simulink model "acc_with_sensor"  (R2021b)
settings: Solver=FixedStepAuto  StartTime=0.0  StopTime=206  FixedStep=0.0005  RelTol=1e-3
InitFcn:
  | G=9.81;
  | m=1660;
  | rw=0.325;
  | Caf=74070;
  | Car=58525;
  | Iz=2778.5;
  | d = 1.502;
  | lf =1.1135;
  | lr =1.5065;
  | L = 2.62;
  | kph2mps=1/3.6;
values from neighbouring files (symbols this model uses):
  Leftdis_PV_switch = 2    [acc_plot_backup.m]
  s_path = [0 1.10508939428 2.2141958029 3.32141571172 4.42705301151 5.53154548532 6.63517443471 7.73808041313 8.84055018688 9.94289959674 11.0453539299 12.1480581097 ... (1001 elements, 1001x1)]    [200_100radius.mat]    (also in LV_Clothoid_S_Turn_path.mat = [0 0.966832089581 1.93621320584 2.90214024471 3.86476766313 ; NEDC_path.mat = [0 0.414605943146 0.832514087334 1.25401518562 1.68216660344; Straight_East_into_curve.mat = [0 1.65770560069 3.32192925577 4.98420060507 6.64484613518 8; acc_plot_backup.m = Station_HV_m)
  X_path = [0 1.10508939428 2.2141958029 3.32141571172 4.42705301151 5.53154548532 6.63517443471 7.73808041313 8.84055018688 9.94289959674 11.0453539299 12.1480581097 ... (1001 elements, 1001x1)]    [200_100radius.mat]    (also in LV_Clothoid_S_Turn_path.mat = [-10 -9.03316791042 -8.06378679416 -7.09785975529 -6.1352323; NEDC_path.mat = [0 0.414605943146 0.832514087334 1.25401518562 1.68216660344; Straight_East_into_curve.mat = [0 1.65770560069 3.32192925577 4.98420060507 6.64484613518 8; acc_plot_backup.m = X_HV_m)
  Y_path = [0 -1.70364610795e-18 -7.41532896709e-18 1.46822109542e-17 4.74557362791e-17 6.12980216762e-17 9.25043977736e-17 1.24088240159e-16 1.5099156923e-16 1.7058517853e-16 1.90629227614e-16 2.09673434424e-16 ... (1001 elements, 1001x1)]    [200_100radius.mat]    (also in LV_Clothoid_S_Turn_path.mat = [0 -8.46153035536e-19 5.07382551045e-18 2.07356032218e-17 3.; NEDC_path.mat = [0 -3.50680326162e-18 -2.14111304971e-18 3.38197671014e-18 3; Straight_East_into_curve.mat = [0 1.29197709199e-18 2.81882429322e-18 3.49020462564e-17 6.7; acc_plot_backup.m = Y_HV_m)
undefined symbols (not defined in the file or in its folder): C_TICK_TIME_S, Cut_in_Secenary_flg, ENUM_ACCSTATE_DISABLED, ENUM_ACCSTATE_OFF, ENUM_ACCSTATE_STANDBY, FALSE, KVDI_ACCLongPressTime_ms, KVDI_ACCMaxActSpeed_kph, KVDI_ACCSetSpdIntial_kph, KVDI_ACCSpdLargeChange_kph, KVDI_LongPressConTime_ms, ONE_FLOAT, ONE_INT, raptor_xcp_function, T, TRUE, UseTTC_switch, ZERO_FLOAT, ZERO_INT
libraries: ADASLibrary x29, simulink x22, Raptor_lib x11, dspstat3 x6, simulink_extras x6, Solver_SF x1, mpclib x1
(part 8 of 9)

== system acc_with_sensor/Relative_Dynamic/Subsystem2/Subsystem ==
  In1 : Inport
  Abs : Abs
  Constant : Constant  Value=0.1
  Switch : Switch  Criteria=u2 > Threshold  Threshold=0.1
  Out1 : Outport
  wires:
  In1/1 -> Switch/1, Abs/1
  Abs/1 -> Switch/2
  Constant/1 -> Switch/3
  Switch/1 -> Out1/1

== system acc_with_sensor/Relative_Dynamic/Subsystem2/Subsystem1 ==
  In1 : Inport
  Abs : Abs
  Constant : Constant  Value=0.1
  Switch : Switch  Criteria=u2 > Threshold  Threshold=0.1
  Out1 : Outport
  wires:
  Switch/1 -> Out1/1
  Constant/1 -> Switch/3
  Abs/1 -> Switch/2
  In1/1 -> Abs/1, Switch/1

== system acc_with_sensor/Relative_Dynamic/Subsystem2/Subsystem2 ==
  In1 : Inport
  Abs : Abs
  Constant : Constant  Value=0.1
  Switch : Switch  Criteria=u2 > Threshold  Threshold=0.1
  Out1 : Outport
  wires:
  In1/1 -> Switch/1, Abs/1
  Abs/1 -> Switch/2
  Constant/1 -> Switch/3
  Switch/1 -> Out1/1

== system acc_with_sensor/Relative_Dynamic/Subsystem2/Subsystem3 ==
  In1 : Inport
  Abs : Abs
  Constant : Constant  Value=0.1
  Switch : Switch  Criteria=u2 > Threshold  Threshold=0.1
  Out1 : Outport
  wires:
  Switch/1 -> Out1/1
  Constant/1 -> Switch/3
  Abs/1 -> Switch/2
  In1/1 -> Abs/1, Switch/1

== system acc_with_sensor/Relative_Dynamic/Subsystem2/acceleration_apr1 ==
  acc_b : Inport
  Abs : Abs
  Constant1 : Constant  Value=0  SampleTime=T
  Switch : Switch  Criteria=u2 > Threshold  Threshold=0.01
  acc_a : Outport  VectorParamsAs1DForOutWhenUnconnected=off
  wires:
  Switch/1 -> acc_a/1
  acc_b/1 -> Abs/1, Switch/1
  Constant1/1 -> Switch/3
  Abs/1 -> Switch/2

== system acc_with_sensor/Relative_Dynamic/Subsystem2/acceleration_apr4 ==
  acc_b : Inport
  Abs : Abs
  Constant1 : Constant  Value=0
  Switch : Switch  Criteria=u2 > Threshold  Threshold=0.01
  acc_a : Outport  VectorParamsAs1DForOutWhenUnconnected=off
  wires:
  Abs/1 -> Switch/2
  Constant1/1 -> Switch/3
  acc_b/1 -> Switch/1, Abs/1
  Switch/1 -> acc_a/1

== system acc_with_sensor/Subsystem2/Subsystem/rolling_avg1 ==
  note: new_average = [ (sample_interval)/(sample_interval + time_constant) ] * (new_value - old_ave) + old_ave
  note: - (FK_TMR/TC)
      |                                    f  =  1  -  e
      |
      |       Where "f" is called the filter constant in the difference equation:
      |
      |                    new_average = f * new_value + (1 - f) * old_average
  note: Using the first two terms of the series expansion:
      |
      |                     x                     x2
      |                                e   =  1  +  x  +  --  + ......
      |                                           2!
      |
      |       Simplifying, the exponential "f" becomes:
      |
      |                  - (FK_TMR/TC)              1
      |           f  =  1  -  e                    =  1  -  -------------  =  . . .
      |                                                    (FK_TMR/TC)
      |                           e
      |
      |                              1                      1
      |          f  =  1  -  ---------------------------------  =    ------------------- .
      |                                  1 + (FK_TMR / TC)       1 + (TC / FK_TMR)
  new_value : Inport
  old_ave : Inport  Port=2
  delta_t : Inport  Port=3
  tc : Inport  Port=4
  Divide : Product  Inputs=*/
  IC : UnitDelay  Tag=struct('comment',struct('text','','placement',1),'logdata',struct('maxnumvals',inf,'plotchannels',[],'stepsize',0,'downsampling',1,'loggingmode',3,'channels',1),'output',struct('width',1,'name','$S_$B','unit','','type','Int16','offset',0,'max',NaN,'min',NaN,'freeze',1,'lsb',1,'arb',0,'class','default','address','','description','','autoscalingmode',1,'lowerheadroom',1,'upperheadroom',1,'headroomunit','bit','checkmin',0,'checkmax',0,'show',0,'initial','2'),'state',0,'dt','-1','date',731455.586925799)  InitialCondition=1  SampleTime=T  HasFrameUpgradeWarning=on
  Interval Test : simulink/Logic and Bit Operations/Interval Test  IntervalClosedRight=on  uplimit=0.00001  IntervalClosedLeft=on  lowlimit=-0.00001  OutDataTypeStr=boolean
  Logical Operator : Logic  Operator=NOT  AllPortsSameDT=off  OutDataTypeStr=boolean
  Product_tmp1 : Product  Tag=struct('comment',struct('text','','placement',1),'logdata',struct('maxnumvals',inf,'plotchannels',[],'stepsize',0,'downsampling',1,'loggingmode',3,'channels',1),'output',struct('width',1,'name','$S_$B','unit','','type','Int32Bin15','offset',0,'max',65535,'min',-65536,'freeze',1,'lsb',2^-15,'arb',0,'class','default','address','','description','','autoscalingmode',1,'lowerheadroom',1,'upperheadroom',1,'headroomunit','bit','checkmin',0,'checkmax',0,'show',0),'inputs','**','exceptionhandling',1,'date',731455.58640515)  Inputs=**  InputSameDT=on  RndMeth=Zero  OutDataTypeStr=Inherit: Same as first input
  Sum : Sum  Tag=struct('comment',struct('text','','placement',1),'logdata',struct('maxnumvals',inf,'plotchannels',[],'stepsize',0,'downsampling',1,'loggingmode',3,'channels',1),'output',struct('width',1,'name','$S_$B','unit','','type','Int32Bin15','offset',0,'max',65535,'min',-65536,'freeze',1,'lsb',2^-15,'arb',0,'class','default','address','','description','','autoscalingmode',1,'lowerheadroom',1,'upperheadroom',1,'headroomunit','bit','checkmin',0,'checkmax',0,'show',0),'inputs','-+','date',731455.586330463)  Inputs=-+  InputSameDT=on  OutDataTypeStr=Inherit: Same as first input
  Sum1 : Sum  Tag=struct('comment',struct('text','','placement',1),'logdata',struct('maxnumvals',inf,'plotchannels',[],'stepsize',0,'downsampling',1,'loggingmode',3,'channels',1),'output',struct('width',1,'name','$S_$B','unit','','type','Int32Bin15','offset',0,'max',65535,'min',-65536,'freeze',1,'lsb',2^-15,'arb',0,'class','default','address','','description','','autoscalingmode',1,'lowerheadroom',1,'upperheadroom',1,'headroomunit','bit','checkmin',0,'checkmax',0,'show',0),'inputs','++','date',731455.58628235)  InputSameDT=on  OutDataTypeStr=Inherit: Same as first input
  Sum2 : Sum  Tag=struct('comment',struct('text','','placement',1),'logdata',struct('maxnumvals',inf,'plotchannels',[],'stepsize',0,'downsampling',1,'loggingmode',3,'channels',1),'output',struct('width',1,'name','$S_$B','unit','','type','Int32Bin15','offset',0,'max',65535,'min',-65536,'freeze',1,'lsb',2^-15,'arb',0,'class','default','address','','description','','autoscalingmode',1,'lowerheadroom',1,'upperheadroom',1,'headroomunit','bit','checkmin',0,'checkmax',0,'show',0),'inputs','++','date',731455.586506424)  InputSameDT=on  OutDataTypeStr=Inherit: Same as first input
  Switch : Switch  Criteria=u2 ~= 0
  Switch1 : Switch  Tag=struct('comment',struct('text','','placement',1),'logdata',struct('maxnumvals',inf,'plotchannels',[],'stepsize',0,'downsampling',1,'loggingmode',3,'channels',1),'output',struct('width',1,'name','$S_$B','unit','','type','Int32Bin15','offset',0,'max',65535,'min',-65536,'freeze',1,'lsb',2^-15,'arb',0,'class','default','address','','description','','autoscalingmode',1,'lowerheadroom',1,'upperheadroom',1,'headroomunit','bit','checkmin',0,'checkmax',0,'show',0),'threshold',struct('width',1,'name','$S_$B_threshold','unit','','type','Int16','offset',0,'max',NaN,'min',NaN,'freeze',1,'lsb',1,'arb',0,'class','default','address','','description','','value','1','scalar',0),'date',731455.58657044)  Threshold=0.5  InputSameDT=on
  zero : Constant  Tag=struct('comment',struct('text','','placement',1),'output',struct('width',1,'name','$S_$B','unit','','type','Int16','offset',0,'max',NaN,'min',NaN,'freeze',1,'lsb',1,'arb',0,'class','default','address','','description','','value','0','tolerance',1,'show',0),'date',731455.58675544)  Value=0  OutDataTypeStr=Inherit: Inherit via back propagation
  zero1 : Constant  Tag=struct('comment',struct('text','','placement',1),'output',struct('width',1,'name','$S_$B','unit','','type','Int16','offset',0,'max',NaN,'min',NaN,'freeze',1,'lsb',1,'arb',0,'class','default','address','','description','','value','0','tolerance',1,'show',0),'date',731455.58675544)  Value=0  OutDataTypeStr=Inherit: Inherit via back propagation
  new_ave : Outport
  wires:
  Switch/1 -> Sum2/2
  Product_tmp1/1 -> Divide/1
  [new_value] -> Switch1/1
  Sum2/1 -> Switch1/3  "new_ave"
  new_value/1 -> [new_value], Sum/2  "new_value"
  Switch1/1 -> new_ave/1  "new_ave"
  Sum/1 -> Product_tmp1/1
  tc/1 -> Sum1/2
  delta_t/1 -> Sum1/1, Product_tmp1/2  "delta_t"
  zero/1 -> IC/1
  old_ave/1 -> Sum/1, Sum2/1  "old_ave"
  Sum1/1 -> Interval Test/1, Divide/2
  zero1/1 -> Switch/3
  Interval Test/1 -> Logical Operator/1
  Divide/1 -> Switch/1
  Logical Operator/1 -> Switch/2
  IC/1 -> Switch1/2

== system acc_with_sensor/Subsystem2/Subsystem1/rolling_avg1 ==
  note: Using the first two terms of the series expansion:
      |
      |                     x                     x2
      |                                e   =  1  +  x  +  --  + ......
      |                                           2!
      |
      |       Simplifying, the exponential "f" becomes:
      |
      |                  - (FK_TMR/TC)              1
      |           f  =  1  -  e                    =  1  -  -------------  =  . . .
      |                                                    (FK_TMR/TC)
      |                           e
      |
      |                              1                      1
      |          f  =  1  -  ---------------------------------  =    ------------------- .
      |                                  1 + (FK_TMR / TC)       1 + (TC / FK_TMR)
  note: - (FK_TMR/TC)
      |                                    f  =  1  -  e
      |
      |       Where "f" is called the filter constant in the difference equation:
      |
      |                    new_average = f * new_value + (1 - f) * old_average
  note: new_average = [ (sample_interval)/(sample_interval + time_constant) ] * (new_value - old_ave) + old_ave
  new_value : Inport
  old_ave : Inport  Port=2
  delta_t : Inport  Port=3
  tc : Inport  Port=4
  Divide : Product  Inputs=*/
  IC : UnitDelay  Tag=struct('comment',struct('text','','placement',1),'logdata',struct('maxnumvals',inf,'plotchannels',[],'stepsize',0,'downsampling',1,'loggingmode',3,'channels',1),'output',struct('width',1,'name','$S_$B','unit','','type','Int16','offset',0,'max',NaN,'min',NaN,'freeze',1,'lsb',1,'arb',0,'class','default','address','','description','','autoscalingmode',1,'lowerheadroom',1,'upperheadroom',1,'headroomunit','bit','checkmin',0,'checkmax',0,'show',0,'initial','2'),'state',0,'dt','-1','date',731455.586925799)  InitialCondition=1  SampleTime=T  HasFrameUpgradeWarning=on
  Interval Test : simulink/Logic and Bit Operations/Interval Test  IntervalClosedRight=on  uplimit=0.00001  IntervalClosedLeft=on  lowlimit=-0.00001  OutDataTypeStr=boolean
  Logical Operator : Logic  Operator=NOT  AllPortsSameDT=off  OutDataTypeStr=boolean
  Product_tmp1 : Product  Tag=struct('comment',struct('text','','placement',1),'logdata',struct('maxnumvals',inf,'plotchannels',[],'stepsize',0,'downsampling',1,'loggingmode',3,'channels',1),'output',struct('width',1,'name','$S_$B','unit','','type','Int32Bin15','offset',0,'max',65535,'min',-65536,'freeze',1,'lsb',2^-15,'arb',0,'class','default','address','','description','','autoscalingmode',1,'lowerheadroom',1,'upperheadroom',1,'headroomunit','bit','checkmin',0,'checkmax',0,'show',0),'inputs','**','exceptionhandling',1,'date',731455.58640515)  Inputs=**  InputSameDT=on  RndMeth=Zero  OutDataTypeStr=Inherit: Same as first input
  Sum : Sum  Tag=struct('comment',struct('text','','placement',1),'logdata',struct('maxnumvals',inf,'plotchannels',[],'stepsize',0,'downsampling',1,'loggingmode',3,'channels',1),'output',struct('width',1,'name','$S_$B','unit','','type','Int32Bin15','offset',0,'max',65535,'min',-65536,'freeze',1,'lsb',2^-15,'arb',0,'class','default','address','','description','','autoscalingmode',1,'lowerheadroom',1,'upperheadroom',1,'headroomunit','bit','checkmin',0,'checkmax',0,'show',0),'inputs','-+','date',731455.586330463)  Inputs=-+  InputSameDT=on  OutDataTypeStr=Inherit: Same as first input
  Sum1 : Sum  Tag=struct('comment',struct('text','','placement',1),'logdata',struct('maxnumvals',inf,'plotchannels',[],'stepsize',0,'downsampling',1,'loggingmode',3,'channels',1),'output',struct('width',1,'name','$S_$B','unit','','type','Int32Bin15','offset',0,'max',65535,'min',-65536,'freeze',1,'lsb',2^-15,'arb',0,'class','default','address','','description','','autoscalingmode',1,'lowerheadroom',1,'upperheadroom',1,'headroomunit','bit','checkmin',0,'checkmax',0,'show',0),'inputs','++','date',731455.58628235)  InputSameDT=on  OutDataTypeStr=Inherit: Same as first input
  Sum2 : Sum  Tag=struct('comment',struct('text','','placement',1),'logdata',struct('maxnumvals',inf,'plotchannels',[],'stepsize',0,'downsampling',1,'loggingmode',3,'channels',1),'output',struct('width',1,'name','$S_$B','unit','','type','Int32Bin15','offset',0,'max',65535,'min',-65536,'freeze',1,'lsb',2^-15,'arb',0,'class','default','address','','description','','autoscalingmode',1,'lowerheadroom',1,'upperheadroom',1,'headroomunit','bit','checkmin',0,'checkmax',0,'show',0),'inputs','++','date',731455.586506424)  InputSameDT=on  OutDataTypeStr=Inherit: Same as first input
  Switch : Switch  Criteria=u2 ~= 0
  Switch1 : Switch  Tag=struct('comment',struct('text','','placement',1),'logdata',struct('maxnumvals',inf,'plotchannels',[],'stepsize',0,'downsampling',1,'loggingmode',3,'channels',1),'output',struct('width',1,'name','$S_$B','unit','','type','Int32Bin15','offset',0,'max',65535,'min',-65536,'freeze',1,'lsb',2^-15,'arb',0,'class','default','address','','description','','autoscalingmode',1,'lowerheadroom',1,'upperheadroom',1,'headroomunit','bit','checkmin',0,'checkmax',0,'show',0),'threshold',struct('width',1,'name','$S_$B_threshold','unit','','type','Int16','offset',0,'max',NaN,'min',NaN,'freeze',1,'lsb',1,'arb',0,'class','default','address','','description','','value','1','scalar',0),'date',731455.58657044)  Threshold=0.5  InputSameDT=on
  zero : Constant  Tag=struct('comment',struct('text','','placement',1),'output',struct('width',1,'name','$S_$B','unit','','type','Int16','offset',0,'max',NaN,'min',NaN,'freeze',1,'lsb',1,'arb',0,'class','default','address','','description','','value','0','tolerance',1,'show',0),'date',731455.58675544)  Value=0  OutDataTypeStr=Inherit: Inherit via back propagation
  zero1 : Constant  Tag=struct('comment',struct('text','','placement',1),'output',struct('width',1,'name','$S_$B','unit','','type','Int16','offset',0,'max',NaN,'min',NaN,'freeze',1,'lsb',1,'arb',0,'class','default','address','','description','','value','0','tolerance',1,'show',0),'date',731455.58675544)  Value=0  OutDataTypeStr=Inherit: Inherit via back propagation
  new_ave : Outport
  wires:
  IC/1 -> Switch1/2
  Logical Operator/1 -> Switch/2
  Divide/1 -> Switch/1
  Interval Test/1 -> Logical Operator/1
  zero1/1 -> Switch/3
  Sum1/1 -> Divide/2, Interval Test/1
  old_ave/1 -> Sum2/1, Sum/1  "old_ave"
  zero/1 -> IC/1
  delta_t/1 -> Product_tmp1/2, Sum1/1  "delta_t"
  tc/1 -> Sum1/2
  Sum/1 -> Product_tmp1/1
  Switch1/1 -> new_ave/1  "new_ave"
  new_value/1 -> Sum/2, [new_value]  "new_value"
  Sum2/1 -> Switch1/3  "new_ave"
  [new_value] -> Switch1/1
  Product_tmp1/1 -> Divide/1
  Switch/1 -> Sum2/2

== system acc_with_sensor/Subsystem22/cmd_limiter1/rate_limit ==
  input_raw : Inport
  Sample_Time : Inport  Port=2
  ratelimt_incps : Inport  Port=3
  ratelimt_decps : Inport  Port=4
  Add : Sum  Inputs=+-
  Add1 : Sum
  Constant : Constant  Value=0  SampleTime=T
  Max : MinMax  Function=max  Inputs=2
  Max1 : MinMax  Inputs=2
  Max2 : MinMax  Function=max  Inputs=2
  Max3 : MinMax  Inputs=2
  Product : Product
  Product1 : Product
  Unit Delay : UnitDelay  SampleTime=T  HasFrameUpgradeWarning=on
  ax_cmd1 : Outport
  wires:
  input_raw/1 -> Add/1
  Add/1 -> Max/1
  Max/1 -> Max1/2
  [Inc] -> Max1/1
  [Dec] -> Max/2
  Max1/1 -> Add1/1
  Add1/1 -> Unit Delay/1, ax_cmd1/1
  Unit Delay/1 -> Add/2, Add1/2
  Max2/1 -> [Inc]
  Max3/1 -> [Dec]
  Constant/1 -> Max3/1, Max2/2
  ratelimt_decps/1 -> Product/2
  ratelimt_incps/1 -> Product1/1
  Sample_Time/1 -> Product1/2, Product/1
  Product/1 -> Max3/2
  Product1/1 -> Max2/1

== system acc_with_sensor/Subsystem22/cmd_limiter2/rate_limit ==
  input_raw : Inport
  Sample_Time : Inport  Port=2
  ratelimt_incps : Inport  Port=3
  ratelimt_decps : Inport  Port=4
  Add : Sum  Inputs=+-
  Add1 : Sum
  Constant : Constant  Value=0  SampleTime=T
  Max : MinMax  Function=max  Inputs=2
  Max1 : MinMax  Inputs=2
  Max2 : MinMax  Function=max  Inputs=2
  Max3 : MinMax  Inputs=2
  Product : Product
  Product1 : Product
  Unit Delay : UnitDelay  SampleTime=T  HasFrameUpgradeWarning=on
  ax_cmd1 : Outport
  wires:
  Product1/1 -> Max2/1
  Product/1 -> Max3/2
  Sample_Time/1 -> Product/1, Product1/2
  ratelimt_incps/1 -> Product1/1
  ratelimt_decps/1 -> Product/2
  Constant/1 -> Max2/2, Max3/1
  Max3/1 -> [Dec]
  Max2/1 -> [Inc]
  Unit Delay/1 -> Add1/2, Add/2
  Add1/1 -> ax_cmd1/1, Unit Delay/1
  Max1/1 -> Add1/1
  [Dec] -> Max/2
  [Inc] -> Max1/1
  Max/1 -> Max1/2
  Add/1 -> Max/1
  input_raw/1 -> Add/1

== system acc_with_sensor/Subsystem5/Lat_selector1/Latch ==
  set : Inport
  reset : Inport  Port=2
  Delay : Delay  DelayLength=1
  Logical Operator3 : Logic  AllPortsSameDT=off  OutDataTypeStr=boolean
  Logical Operator4 : Logic  Operator=NOT  AllPortsSameDT=off  OutDataTypeStr=boolean
  Switch : Switch  Criteria=u2 ~= 0
  Switch1 : Switch  Criteria=u2 ~= 0
  latched : Outport
  wires:
  Delay/1 -> Switch1/3
  Logical Operator4/1 -> Logical Operator3/2, Switch1/1
  Logical Operator3/1 -> Switch/2
  reset/1 -> Logical Operator4/1, Switch1/2
  Switch/1 -> Delay/1, latched/1
  set/1 -> Switch/1, Logical Operator3/1
  Switch1/1 -> Switch/3

== system acc_with_sensor/Subsystem5/Lat_selector1/Smooth Switch1 ==
  Dynamic_cmd : Inport
  Mode : Inport  Port=2
  Kinematic_cmd : Inport  Port=3
  Add12 : Sum
  Add9 : Sum  Inputs=+-
  Constant : Constant  SampleTime=T
  Constant1 : Constant  Value=0  SampleTime=T
  Constant49 : Constant  SampleTime=T
  Data Type Conversion : DataTypeConversion  OutDataTypeStr=double
  Limit : ADASLibrary/Limit  SystemSampleTime=-1  VariantActivationTime=update diagram  Latency=0  AutoFrameSizeCalculation=off
      settings: SourceProductName=ADASLibrary
  Product1 : Product
  Product2 : Product
  ax_cmd : Outport
  wires:
  Mode/1 -> Data Type Conversion/1
  Add12/1 -> ax_cmd/1
  Add9/1 -> Product1/1
  Kinematic_cmd/1 -> Product1/2
  Product1/1 -> Add12/2
  Constant49/1 -> Add9/1
  Limit/1 -> Product2/2, Add9/2
  Dynamic_cmd/1 -> Product2/1
  Product2/1 -> Add12/1
  Data Type Conversion/1 -> Limit/1
  Constant/1 -> Limit/2
  Constant1/1 -> Limit/3

== system acc_with_sensor/Subsystem5/Lat_selector1/Subsystem ==
  new_value : Inport
  Constant83 : Constant  Value=0.3  SampleTime=T
  Constant84 : Constant  Value=0.1  SampleTime=T
  Delay11 : Delay  DelayLength=1  SampleTime=T
  rolling_avg1 : Subsystem
  new_ave : Outport
  wires:
  Delay11/1 -> rolling_avg1/2(old_ave)
  Constant84/1 -> rolling_avg1/3(delta_t)  "T"
  Constant83/1 -> rolling_avg1/4(tc)
  rolling_avg1/1(new_ave) -> Delay11/1, new_ave/1
  new_value/1 -> rolling_avg1/1(new_value)

== system acc_with_sensor/Subsystem5/MPC_Dynematc1/R selector ==
  LaneAvail_fig : Inport
  vx : Inport  Port=2
  1-D Lookup Table2 : Lookup_n-D  NumberOfTableDimensions=1  BreakpointsForDimension1=[0 15 28 40]/3.6  Table=[31 31 35 35]  InternalRulePriority=Speed  RndMeth=Simplest  InputSameDT=on
  Constant1 : Constant  Value=35
  Constant19 : Constant
  Constant2 : Constant  Value=20
  Constant66 : Constant  Value=0.5  SampleTime=T
  Switch12 : Switch  Criteria=u2 > Threshold
  R : Outport
  wires:
  vx/1 -> 1-D Lookup Table2/1
  Switch12/1 -> R/1
  LaneAvail_fig/1 -> Switch12/2
  1-D Lookup Table2/1 -> Switch12/3
  Constant66/1 -> Switch12/1

== system acc_with_sensor/Subsystem5/MPC_Dynematc2/R selector1 ==
  LaneAvail_flg : Inport
  vx : Inport  Port=2
  1-D Lookup Table2 : Lookup_n-D  Commented=on  NumberOfTableDimensions=1  BreakpointsForDimension1=[0 15 28 40]/3.6  Table=[31 31 35 35]  InternalRulePriority=Speed  RndMeth=Simplest  InputSameDT=on
  Constant1 : Constant  Value=35
  Constant19 : Constant
  Constant2 : Constant  Value=7
  Constant66 : Constant  Value=0.5
  Switch12 : Switch  Criteria=u2 > Threshold
  R_D : Outport
  wires:
  Switch12/1 -> R_D/1
  LaneAvail_flg/1 -> Switch12/2
  Constant2/1 -> Switch12/3
  Constant66/1 -> Switch12/1

== system acc_with_sensor/Subsystem8/cmd_limiter1/rate_limit ==
  input_raw : Inport
  Sample_Time : Inport  Port=2
  ratelimt_incps : Inport  Port=3
  ratelimt_decps : Inport  Port=4
  Add : Sum  Inputs=+-
  Add1 : Sum
  Constant : Constant  Value=0  SampleTime=T
  Max : MinMax  Function=max  Inputs=2
  Max1 : MinMax  Inputs=2
  Max2 : MinMax  Function=max  Inputs=2
  Max3 : MinMax  Inputs=2
  Product : Product
  Product1 : Product
  Unit Delay : UnitDelay  SampleTime=T  HasFrameUpgradeWarning=on
  ax_cmd1 : Outport
  wires:
  input_raw/1 -> Add/1
  Add/1 -> Max/1
  Max/1 -> Max1/2
  [Inc] -> Max1/1
  [Dec] -> Max/2
  Max1/1 -> Add1/1
  Add1/1 -> Unit Delay/1, ax_cmd1/1
  Unit Delay/1 -> Add/2, Add1/2
  Max2/1 -> [Inc]
  Max3/1 -> [Dec]
  Constant/1 -> Max3/1, Max2/2
  ratelimt_decps/1 -> Product/2
  ratelimt_incps/1 -> Product1/1
  Sample_Time/1 -> Product1/2, Product/1
  Product/1 -> Max3/2
  Product1/1 -> Max2/1

== system acc_with_sensor/Subsystem8/cmd_limiter2/rate_limit ==
  input_raw : Inport
  Sample_Time : Inport  Port=2
  ratelimt_incps : Inport  Port=3
  ratelimt_decps : Inport  Port=4
  Add : Sum  Inputs=+-
  Add1 : Sum
  Constant : Constant  Value=0  SampleTime=T
  Max : MinMax  Function=max  Inputs=2
  Max1 : MinMax  Inputs=2
  Max2 : MinMax  Function=max  Inputs=2
  Max3 : MinMax  Inputs=2
  Product : Product
  Product1 : Product
  Unit Delay : UnitDelay  SampleTime=T  HasFrameUpgradeWarning=on
  ax_cmd1 : Outport
  wires:
  Product1/1 -> Max2/1
  Product/1 -> Max3/2
  Sample_Time/1 -> Product/1, Product1/2
  ratelimt_incps/1 -> Product1/1
  ratelimt_decps/1 -> Product/2
  Constant/1 -> Max2/2, Max3/1
  Max3/1 -> [Dec]
  Max2/1 -> [Inc]
  Unit Delay/1 -> Add1/2, Add/2
  Add1/1 -> ax_cmd1/1, Unit Delay/1
  Max1/1 -> Add1/1
  [Dec] -> Max/2
  [Inc] -> Max1/1
  Max/1 -> Max1/2
  Add/1 -> Max/1
  input_raw/1 -> Add/1

== system acc_with_sensor/Subsystem5/Lat_selector1/Subsystem/rolling_avg1 ==
  note: Using the first two terms of the series expansion:
      |
      |                     x                     x2
      |                                e   =  1  +  x  +  --  + ......
      |                                           2!
      |
      |       Simplifying, the exponential "f" becomes:
      |
      |                  - (FK_TMR/TC)              1
      |           f  =  1  -  e                    =  1  -  -------------  =  . . .
      |                                                    (FK_TMR/TC)
      |                           e
      |
      |                              1                      1
      |          f  =  1  -  ---------------------------------  =    ------------------- .
      |                                  1 + (FK_TMR / TC)       1 + (TC / FK_TMR)
  note: - (FK_TMR/TC)
      |                                    f  =  1  -  e
      |
      |       Where "f" is called the filter constant in the difference equation:
      |
      |                    new_average = f * new_value + (1 - f) * old_average
  note: new_average = [ (sample_interval)/(sample_interval + time_constant) ] * (new_value - old_ave) + old_ave
  new_value : Inport
  old_ave : Inport  Port=2
  delta_t : Inport  Port=3
  tc : Inport  Port=4
  Divide : Product  Inputs=*/
  IC : UnitDelay  Tag=struct('comment',struct('text','','placement',1),'logdata',struct('maxnumvals',inf,'plotchannels',[],'stepsize',0,'downsampling',1,'loggingmode',3,'channels',1),'output',struct('width',1,'name','$S_$B','unit','','type','Int16','offset',0,'max',NaN,'min',NaN,'freeze',1,'lsb',1,'arb',0,'class','default','address','','description','','autoscalingmode',1,'lowerheadroom',1,'upperheadroom',1,'headroomunit','bit','checkmin',0,'checkmax',0,'show',0,'initial','2'),'state',0,'dt','-1','date',731455.586925799)  InitialCondition=1  SampleTime=T  HasFrameUpgradeWarning=on
  Interval Test : simulink/Logic and Bit Operations/Interval Test  IntervalClosedRight=on  uplimit=0.00001  IntervalClosedLeft=on  lowlimit=-0.00001  OutDataTypeStr=boolean
  Logical Operator : Logic  Operator=NOT  AllPortsSameDT=off  OutDataTypeStr=boolean
  Product_tmp1 : Product  Tag=struct('comment',struct('text','','placement',1),'logdata',struct('maxnumvals',inf,'plotchannels',[],'stepsize',0,'downsampling',1,'loggingmode',3,'channels',1),'output',struct('width',1,'name','$S_$B','unit','','type','Int32Bin15','offset',0,'max',65535,'min',-65536,'freeze',1,'lsb',2^-15,'arb',0,'class','default','address','','description','','autoscalingmode',1,'lowerheadroom',1,'upperheadroom',1,'headroomunit','bit','checkmin',0,'checkmax',0,'show',0),'inputs','**','exceptionhandling',1,'date',731455.58640515)  Inputs=**  InputSameDT=on  RndMeth=Zero  OutDataTypeStr=Inherit: Same as first input
  Sum : Sum  Tag=struct('comment',struct('text','','placement',1),'logdata',struct('maxnumvals',inf,'plotchannels',[],'stepsize',0,'downsampling',1,'loggingmode',3,'channels',1),'output',struct('width',1,'name','$S_$B','unit','','type','Int32Bin15','offset',0,'max',65535,'min',-65536,'freeze',1,'lsb',2^-15,'arb',0,'class','default','address','','description','','autoscalingmode',1,'lowerheadroom',1,'upperheadroom',1,'headroomunit','bit','checkmin',0,'checkmax',0,'show',0),'inputs','-+','date',731455.586330463)  Inputs=-+  InputSameDT=on  OutDataTypeStr=Inherit: Same as first input
  Sum1 : Sum  Tag=struct('comment',struct('text','','placement',1),'logdata',struct('maxnumvals',inf,'plotchannels',[],'stepsize',0,'downsampling',1,'loggingmode',3,'channels',1),'output',struct('width',1,'name','$S_$B','unit','','type','Int32Bin15','offset',0,'max',65535,'min',-65536,'freeze',1,'lsb',2^-15,'arb',0,'class','default','address','','description','','autoscalingmode',1,'lowerheadroom',1,'upperheadroom',1,'headroomunit','bit','checkmin',0,'checkmax',0,'show',0),'inputs','++','date',731455.58628235)  InputSameDT=on  OutDataTypeStr=Inherit: Same as first input
  Sum2 : Sum  Tag=struct('comment',struct('text','','placement',1),'logdata',struct('maxnumvals',inf,'plotchannels',[],'stepsize',0,'downsampling',1,'loggingmode',3,'channels',1),'output',struct('width',1,'name','$S_$B','unit','','type','Int32Bin15','offset',0,'max',65535,'min',-65536,'freeze',1,'lsb',2^-15,'arb',0,'class','default','address','','description','','autoscalingmode',1,'lowerheadroom',1,'upperheadroom',1,'headroomunit','bit','checkmin',0,'checkmax',0,'show',0),'inputs','++','date',731455.586506424)  InputSameDT=on  OutDataTypeStr=Inherit: Same as first input
  Switch : Switch  Criteria=u2 ~= 0
  Switch1 : Switch  Tag=struct('comment',struct('text','','placement',1),'logdata',struct('maxnumvals',inf,'plotchannels',[],'stepsize',0,'downsampling',1,'loggingmode',3,'channels',1),'output',struct('width',1,'name','$S_$B','unit','','type','Int32Bin15','offset',0,'max',65535,'min',-65536,'freeze',1,'lsb',2^-15,'arb',0,'class','default','address','','description','','autoscalingmode',1,'lowerheadroom',1,'upperheadroom',1,'headroomunit','bit','checkmin',0,'checkmax',0,'show',0),'threshold',struct('width',1,'name','$S_$B_threshold','unit','','type','Int16','offset',0,'max',NaN,'min',NaN,'freeze',1,'lsb',1,'arb',0,'class','default','address','','description','','value','1','scalar',0),'date',731455.58657044)  Threshold=0.5  InputSameDT=on
  zero : Constant  Tag=struct('comment',struct('text','','placement',1),'output',struct('width',1,'name','$S_$B','unit','','type','Int16','offset',0,'max',NaN,'min',NaN,'freeze',1,'lsb',1,'arb',0,'class','default','address','','description','','value','0','tolerance',1,'show',0),'date',731455.58675544)  Value=0  OutDataTypeStr=Inherit: Inherit via back propagation
  zero1 : Constant  Tag=struct('comment',struct('text','','placement',1),'output',struct('width',1,'name','$S_$B','unit','','type','Int16','offset',0,'max',NaN,'min',NaN,'freeze',1,'lsb',1,'arb',0,'class','default','address','','description','','value','0','tolerance',1,'show',0),'date',731455.58675544)  Value=0  OutDataTypeStr=Inherit: Inherit via back propagation  SampleTime=T
  new_ave : Outport
  wires:
  IC/1 -> Switch1/2
  Logical Operator/1 -> Switch/2
  Divide/1 -> Switch/1
  Interval Test/1 -> Logical Operator/1
  zero1/1 -> Switch/3
  Sum1/1 -> Divide/2, Interval Test/1
  old_ave/1 -> Sum2/1, Sum/1  "old_ave"
  zero/1 -> IC/1
  delta_t/1 -> Product_tmp1/2, Sum1/1  "delta_t"
  tc/1 -> Sum1/2
  Sum/1 -> Product_tmp1/1
  Switch1/1 -> new_ave/1  "new_ave"
  new_value/1 -> Sum/2, [new_value]  "new_value"
  Sum2/1 -> Switch1/3  "new_ave"
  [new_value] -> Switch1/1
  Product_tmp1/1 -> Divide/1
  Switch/1 -> Sum2/2

== matlab function acc_with_sensor/MPC_ACC1 ==
  data: D_rel input; A output; V_rel input; ax_rel input; B output; C output; Yref output; x_state output; vx input; ACCSetSpeed_mps input; ax input; Desired_dist output
function [A,B,C,Yref,x_state,Desired_dist]   = fcn(D_rel,V_rel,ax_rel,vx,ACCSetSpeed_mps,ax)

% Parameter
T=0.1;
tau=0.3;

% Model
 A = [1 T 0.5*T^2;
          0 1 T;
          0 0 1-T/tau];
% A = [1 T 0;
%          0 1 T;
%          0 0 1-T/tau];
B = [0;0;T/tau];
C = [1 0 0];

x_state =[D_rel-2;V_rel;ax_rel];

Yref=zeros(10,1);
Vx=min([vx ACCSetSpeed_mps]);
for i=1:10
    Yref(i)=1.5*((ax*0.1*(i-1)+Vx));
%     if Yref_TH(i)<=0
%         Yref_TH(i)=0;
%     end
end

Desired_dist=Yref(1)+2;

end

== matlab function acc_with_sensor/Subsystem7/MPC_ACC4 ==
  data: A input; B input; C input; Yref input; x_state input; Np input; Nc input; u output size=1; Qs input; Rs input; u_old input
function u  = fcn(A,B,C,Yref,x_state,Np,Nc,Qs,Rs,u_old)

[m_A,n_A] = size(A);

% Delta u version
phi=[A B
    zeros(1,m_A) eye(1)];
gamma=[B;eye(1)];
eta=[C 0];
x=[x_state;u_old];

[m_A,n_A] = size(phi);

F=zeros(Np,m_A);
for i=1:Np
    F(i,:)=eta*(phi^i);
end

K = zeros(Np, Nc);
K(1,1) = eta*gamma;
K(2:Np,1) = F(1:Np-1,:)*gamma;
for k = 2:Nc
K(:,k) =circshift(K(:,1),k-1);
end
K = tril(K);

Q=Qs.*eye(Np); %Qw權重值=1;10
R=Rs.*eye(Nc);%Rw權重值=0.07;1.5 ,0.07


H = K'*Q*K+R;
f = K'*Q*(Yref-F*x);
U = H\f;
u = U(1)+u_old;

end

== matlab function acc_with_sensor/V_rel Estimation/Kalman filter/MATLAB Function2 ==
  data: X1 input; X2 output; K input; Y input
function X2 = fcn(X1,K,Y)%Y=相對速度
H=[1 0 0];
X2=X1+K*(Y-H*X1);
end

== matlab function acc_with_sensor/V_rel Estimation/Kalman filter/measurement update ==
  data: X2 input; u input; X1 output
function X1 = fcn(X2,u)%u=jerk input
T=0.1;
F=[1 T 0.5*T^2;0 1 T;0 0 1];
G=[-1/6*T^3;-1/2*T^2;-T];
X1=F*X2+G*u;
end

== matlab function acc_with_sensor/V_rel Estimation/Kalman filter/time update ==
  data: Q input; K output; R input; M1 input; M2 output
function [K,M2] = fcn(Q,R,M1)
T=0.1;%sample time
F=[1 T 0.5*T^2;0 1 T;0 0 1];%system matrix
H=[1 0 0];%output matrix
G=[-(T^3)/6;-(T^2)/2;-T];%
%誤差斜方矩陣
P=M1-M1*H'*inv(H*M1*H'+R)*H*M1;
M2=F*P*F'+G*Q*G';
K=P*H'*inv(R);
end

== matlab function acc_with_sensor/Acceleration controller2 ==
  data: axc input; Tr output; Vxh input; Tb output; Rtotal output; m input
function [Tr,Tb,Rtotal]= fcn(axc, Vxh,m)
% m_hat = 1370+89.9+65.2+22*4; 
m_hat = m;
Cd_hat = 0.3;     %Aerodynamic Coefficient
fr_hat = 0.0038;  %Rolling Resistance Moment

zho = 1.206;  %Air Mass density
Af = 2.2; %Front Area
g = 9.81;
rw = 0.325; %Effective rolling radius 

% m_hat = 1/theta_hat(1);
% Cd_hat = theta_hat(2)*m_hat;
% fr_hat = theta_hat(3);

theta = 0;
% Resistance

Ra = 0.5*zho*Cd_hat*Af*Vxh^2;
Rg = m_hat*g*sin(theta);
Rr = fr_hat*m_hat*g*cos(theta);
Rtotal = (Ra + Rg + Rr)*rw;

% if Vxh<1
%     Ra=0;
%     Rg=0;
%     Rr=0;
%     Rtotal =0;
% else
%     Ra = 0.5*zho*Cd_hat*Af*Vxh^2;
%     Rg = m_hat*g*sin(theta);
%     Rr = fr_hat*m_hat*g*cos(theta);
%     Rtotal = (Ra + Rg + Rr)*rw;
% end

Tr = (m_hat*axc + Ra + Rg + Rr)*rw;
Tb = (m_hat*axc - Ra - Rg - Rr)*rw;

if axc >= 0
    Tr = Tr;
    Tb = 0;
else
    Tr = 0;
    Tb = Tb;
end

== matlab function acc_with_sensor/MATLAB Function17 ==
  data: trig input; u output; Yref input; tau input; Qs input; Rs input; steer_angle input; Vx input; Ax input; F output
function [u,F]  = fcn( trig,Yref, tau, Qs,Rs,steer_angle,Vx,Ax)
%% parameter
Np=10;
Nc=3;
T = 0.1;

% if case1==1
%    Qs1=8;
%    Rs1=30;
%    Np=35;
% else
%    Qs1=6;
%    Rs1=1;
%    Np=35;
% end



if trig ==1


L=2.650;


Y_ref=Yref(1:Np);


%% vehicle parameter

vx = ones(Np,1)*Vx; %10kph
%     vx=zeros(Np,1);
%     vx(1)=Vx;
%     for z=2:Np
%         vx(z)=vx(z-1)+Ax*T;
%     end
x_state = [0 0 steer_angle]';

%% Vehicle Kinematics Model
A  = [1 vx(1,1)*T vx(1,1)*T;
        0 1 vx(1,1)/L*T;
        0 0 -T/tau+1];
% ----------------------------------------%
% x = [y, yaw angle, steering wheel angle]
% state row =3, state column =3,
%-----------------------------------------%
sr =3;
sc =3;
B = [0 0 (1/tau)*T]';
H = [1 0 0]; % [1, sr]

%% MPC parameter
% ------------------------------------------------------------------------------------------%
% Am is a vertor [A(k); A(k+1); A(k+2) ... A(k+np-1)]
% ------------------------------------------------------------------------------------------%
Am = zeros(sr, sc, Np);
for i = 1 : Np
    Am(:, :, i) = [1 vx(i,1)*T vx(i,1)*T;
                    0 1 vx(i,1)/L*T;
                    0 0 -(T/tau)+1];
end
% ------------------------------------------------------------------------------------------%
% Amm is a vector [A(k); A(k)A(k+1); A(k)A(k+1)A(k+2) ... A(k+np-1)]
% ------------------------------------------------------------------------------------------%
Amm = zeros(sr, sc, Np);
Amm(:, :, 1) = Am(:, :, 1);
for i = 2 : Np
    Amm(:, :, i) = Am(:, :, i) * Amm(:, :, i - 1);
end
% ----------------------------------------------------------------------------------------------%
% F is a metric [H A(k); H A(k)A(k+1); H A(k)A(k+1)A(k+2) ... H A(k+np-1)]
% size = [np, sc]
% ----------------------------------------------------------------------------------------------%
F = zeros(Np, sc);
for i = 1 : Np
    F(i, :) = H * Amm(:, : ,i);
end

% F=zeros(Np,sc);
% for i=1:Np
%     F(i,:)=H*([1 vx(1)*T vx(1)*T;
%                0 1 vx(1)/L*T;
%                0 0 -(T/tau)+1]^Np);
% end

% ----------------------------------------------------------------------------------------------%
% K is a metric [H A(k); H A(k)A(k+1); H A(k)A(k+1)A(k+2) ... H A(k+np-1)]
%size = [np nc]
%[H*B                                 0             0  ...       0  ]
%[H*A(k)*B                       H*B          0  ...        0 ] 
%[H*A(k)*A(k+1)*B       H*A(k)*B      0  ...    H*B ]
% the following quation is modified

%[H*B                                 0                   0          0          ...           0 ]
%[H*A(k+1)*B                          H*B                 0          0          ...           0 ] 
%[H*A(k+2)*A(k+1)*B                 H*A(k+2)*B           H*B         0          ...           0 ]
%[H*A(k+3)*A(k+2)*A(k+1)*B        H*A(k+3)*A(k+2)*B     H*A(k+3)*B   H*B        ...           0 ]
%[H*A(k+np-1)*A(k+np-2)*...*A(k+np-np+1)*B      H*A(k+np-1)*A(k+np-2)*...*A(k+np-np+2)*B     H*A(k+3)*B   H*B        ...           0 ]
% ----------------------------------------------------------------------------------------------%
% K = zeros(Np, Nc);
% K(1,1) = H*B;
% for i = 2 : Np
%     K(i,1) = F(i-1, :) * B;
% end
% for i = 2 : Nc
%     K(i : Np, i) = K(i - 1 : Np - 1, i - 1);
% end
%--------------------------------------------------------------
K = zeros(Np, Nc);
% v = F*B;

v= zeros(Np, 1);

v(1,1) = H*B;
v(2:Np,:) = F(1:Np-1,:)*B;

K(2:Np,1) = v(2:Np,1);
K(1,1) = H*B;


% K(2:Np,1) = v(1:Np-1);
% K(1,1) = H*B;

% K(:,1) = v;

i=0;
for k = 2:Nc
    for kk = k:Np
        i=i+1;
        K(kk,k) = v(i,1); %Toeplitz matrix
    end
    i=0;
end

%% final K
% K = eye(Np, Np);
% K = K * (H*B);
% Kmm = zeros(sr, sc, Np, Np);
% for i = 2 : Np
%     
%     Kmm(:, :, i, i-1) = Am(:, :, i);
%     K(i, i-1) = H * Kmm(:, :, i, i-1) * B;
% end
% 
% r = 1;
% for i = 3 : Np
%     Kmm(:, :, i, 1) = Am(:, :, i) * Kmm(:, :, i-1, 1);
%     K(i, 1) = H * Kmm(:, :, i, 1) * B;
%     m = i;
%     while (m >= 4 && m<=Np)
%         Kmm(:, :, m, r) = Am(:, :, m) * Kmm(:, :, m-1, r);
%         K(m, r) = H * Kmm(:, :, m, r) * B;
%         m = m+1;
%     end
%     r = r+1;
% end
% 
% if Nc ~= Np
%     K = K (1:Np, 1:Nc);
% end

% K = zeros(Np, Nc);
% K(1,1) = H*B;
% for i = 2 : Np
% end

% ----------------------------------------------------------------------------------------------%
%Q is the weighting of reference error
%R is the weighting of control gain
%our object is the minimize the cost function between these two option
% ----------------------------------------------------------------------------------------------%

Q = eye(Np);

Q = Q * Qs;
R = eye(Nc);
R = R * Rs;

% ----------------------------------------------------------------------------------------------%
%cost function
%J = (Rs - Y) * Q * (Rs - Y)' + U * R * U'
% after differential the cost function,and let dJ=0, we can get
%U = inv(K' * Q * K + R) * K' * Q * (rs - F * x_state)
%solve U, and the vector U is the optimal control gain series 

%when Rs == 2
%J = (Rs1 - Y1) * Q1 * (Rs1 - Y1)' + (Rs2 - Y2) * Q2 * (Rs2 - Y2)' + U * R * U'
%U = inv(K1' * Q * K1 + K2' * Q * K2 + R) * (K1' * Q1 * (Rs1 - F1 * x_state) + K2' * Q2 * (Rs2 - F2 * x_state))
% ----------------------------------------------------------------------------------------------%

U = inv(K' * Q * K + R) * K' * Q * (Y_ref - F * x_state);
u=U(1);

else
    u=0;
    F = zeros(Np, 3);
end
end

== matlab function acc_with_sensor/Camera/Subsystem6/Camera_NEW ==
  data: ux_mps input; phi_deg input; Xo input; Yo input; station input; x_ref output size=[22 1]; y_ref output size=[22 1]; Heading_ref output size=[22 1]; C output; Ts_MPC input; X_path input; s_path input; Y_path input
function [x_ref,y_ref,Heading_ref,C]  = Camera_emulator(ux_mps,phi_deg,Xo,Yo, station,Ts_MPC, X_path, s_path, Y_path)
% function [x_ref,y_ref,Y_path,Heading_ref,C]  = Camera_emulator(ux_mps,phi_deg,Xo,Yo, X_path, s_path,station,t_start,Ts_MPC,AES_pre_time,speed,Np,C0_Old, Y_path_Old)
% Path information is X_path, Y_path, s_path 
% Load path before running model===========================================
Np=22;
Tp=Ts_MPC*Np;

phi_rad=phi_deg*pi/180;

% global reference
% Yr=interp1(s_path,Y_path,station);
% path x,y body coordinate=================================================
x_path=cos(phi_rad)*(X_path-Xo)+sin(phi_rad)*(Y_path-Yo);
y_path=-sin(phi_rad)*(X_path-Xo)+cos(phi_rad)*(Y_path-Yo);
% current x,y body coordinate
% x_ref(1)=interp1(s_path,x_path,station);
% y_ref(1)=interp1(s_path,y_path,station);

s=ones(Np+2,1);
delta_s=Ts_MPC*ux_mps;
s=diag(0:Np+1)*s*delta_s+station;
%s=diag(-1:Np)*s*delta_s+station;

x_ref=zeros(Np,1);
y_ref=zeros(Np,1);
x_ref_12=interp1(s_path,x_path,s);
y_ref_12=interp1(s_path,y_path,s);
x_ref=x_ref_12(2:Np+1);
y_ref=y_ref_12(2:Np+1);
s_temp=s(Np)+Ts_MPC*ux_mps;

Heading_ref=zeros(Np,1);

a=zeros(Np,1);
for i=1:Np
    a(i)=x_ref_12(i+2)-x_ref_12(i+1);
    if abs(a(i))<=0.1
        a(i)=0.1;
    end
    Heading_ref(i)=atan2(y_ref_12(i+2)-y_ref_12(i+1),a(i));
end


%% CR=polyfit(x_R,y_R,3);
x=x_ref;
% Lane Change Module ======================================================

% if y_ref >= 1.5
%     y=y_ref-3.66;
% elseif y_ref <= -1.5
%     y=y_ref+3.66;
% else
%     y=y_ref+0;
% end
if y_ref >= 1.5
    y=y_ref-3.66;
elseif y_ref <= -1.5
    y=y_ref+3.66;
else
    y=y_ref+0;
end

%===================================================================
sum_x1=sum(x);
sum_x2=sum(x.^2);
sum_x3=sum(x.^3);
sum_x4=sum(x.^4);
sum_x5=sum(x.^5);
sum_x6=sum(x.^6);
sum_y=sum(y);

% A=[length(x) sum(x) sum(x.^2); sum(x.^3);
%         sum(x) sum(x.^2); sum(x.^3) sum(x.^4); 
%         sum(x.^2); sum(x.^3) sum(x.^4) sum(x.^5); 
%         sum(x.^3) sum(x.^4) sum(x.^5) sum(x.^6)];

% A=[length(x) sum(x) sum(x^2); sum(x^3);
%         sum(x) sum(x^2); sum(x^3) sum(x^4); 
%         sum(x^2); sum(x^3) sum(x^4) sum(x^5); 
%         sum(x^3) sum(x^4) sum(x^5) sum(x^6)];
% sum_x=zeros(Np,1);
% sum_y=zeros(Np,1);
% for r=1:length(Np)
%     sum_x(i)=x(i);
%     sum_y(i)=y(i);
% end

A=[length(x) sum_x1 sum_x2 sum_x3;
    sum_x1 sum_x2 sum_x3 sum_x4; 
    sum_x2 sum_x3 sum_x4 sum_x5; 
    sum_x3 sum_x4 sum_x5 sum_x6];

B=[sum_y;
      sum(x.*y);
      sum(x.*x.*y);
      sum(x.*x.*x.*y)];

% A=eye(4);
% 
% B=[1;
%   1;
%   1;
%   1];

if ux_mps<=0.1
    C=[0; 0; 0; 0];
else
    C=inv(A)*B;
% C=B;
end
end

== matlab function acc_with_sensor/Subsystem/longitudinal_driver_reference ==
  data: longitudinal_lane_refernce_trigger input; T input; Vxo input; Vxt input; ax_max input; jx_max input; Vx output; t output
function [Vx,t] = fcn(longitudinal_lane_refernce_trigger,T,Vxo,Vxt,ax_max,jx_max)
Vx=0;
Ax=0;
t=0;

if Vxt < Vxo
    ax_max=-ax_max;
    jx_max=-jx_max;
end

if longitudinal_lane_refernce_trigger==1

t1=ax_max/jx_max;
t2=(Vxt-Vxo)/ax_max;
t3=t1+t2;
t=T+0.1;


V1=Vxo+(0.5*jx_max*(t1^2));
V2=V1+(ax_max*(t2-t1));
   if t>=0 && t<=t1
       Ax=jx_max*t;
       Vx=double(Vxo+0.5*jx_max*(t^2));
   end
   if t>t1 && t<=t2
       Ax=ax_max;
       Vx=double(V1+(ax_max*(t-t1)));
   end
   if t>t2 && t<=t3
       Ax=ax_max-(jx_max*(t-t2));
       Vx=double(V2+ax_max*(t-t2)-0.5*jx_max*((t-t2)^2));
   end
   if t>t3
       Vx=double(Vxt);
       Ax=0;
   end
       

end
if longitudinal_lane_refernce_trigger==0
  Vx=double(Vxo);
 

   
end
end

== matlab function acc_with_sensor/Subsystem/longitudinal_driver_reference1 ==
  data: longitudinal_lane_refernce_trigger input; T input; Vxo input; Vxt input; ax_max input; jx_max input; Vx output; t output
function [Vx,t] = fcn(longitudinal_lane_refernce_trigger,T,Vxo,Vxt,ax_max,jx_max)
Vx=0;
Ax=0;
t=0;

if Vxt < Vxo
    ax_max=-ax_max;
    jx_max=-jx_max;
end

if longitudinal_lane_refernce_trigger==1

t1=ax_max/jx_max;
t2=(Vxt-Vxo)/ax_max;
t3=t1+t2;
t=T+0.1;


V1=Vxo+(0.5*jx_max*(t1^2));
V2=V1+(ax_max*(t2-t1));
   if t>=0 && t<=t1
       Ax=jx_max*t;
       Vx=double(Vxo+0.5*jx_max*(t^2));
   end
   if t>t1 && t<=t2
       Ax=ax_max;
       Vx=double(V1+(ax_max*(t-t1)));
   end
   if t>t2 && t<=t3
       Ax=ax_max-(jx_max*(t-t2));
       Vx=double(V2+ax_max*(t-t2)-0.5*jx_max*((t-t2)^2));
   end
   if t>t3
       Vx=double(Vxt);
       Ax=0;
   end
       

end
if longitudinal_lane_refernce_trigger==0
  Vx=double(Vxo);
 

   
end
end

== matlab function acc_with_sensor/Subsystem/longitudinal_driver_reference2 ==
  data: longitudinal_lane_refernce_trigger input; T input; Vxo input; Vxt input; ax_max input; jx_max input; Vx output; t output
function [Vx,t] = fcn(longitudinal_lane_refernce_trigger,T,Vxo,Vxt,ax_max,jx_max)
Vx=0;
Ax=0;
t=0;

if Vxt < Vxo
    ax_max=-ax_max;
    jx_max=-jx_max;
end

if longitudinal_lane_refernce_trigger==1

t1=ax_max/jx_max;
t2=(Vxt-Vxo)/ax_max;
t3=t1+t2;
t=T+0.1;


V1=Vxo+(0.5*jx_max*(t1^2));
V2=V1+(ax_max*(t2-t1));
   if t>=0 && t<=t1
       Ax=jx_max*t;
       Vx=double(Vxo+0.5*jx_max*(t^2));
   end
   if t>t1 && t<=t2
       Ax=ax_max;
       Vx=double(V1+(ax_max*(t-t1)));
   end
   if t>t2 && t<=t3
       Ax=ax_max-(jx_max*(t-t2));
       Vx=double(V2+ax_max*(t-t2)-0.5*jx_max*((t-t2)^2));
   end
   if t>t3
       Vx=double(Vxt);
       Ax=0;
   end
       

end
if longitudinal_lane_refernce_trigger==0
  Vx=double(Vxo);
 

   
end
end

== matlab function acc_with_sensor/Subsystem/longitudinal_driver_reference3 ==
  data: longitudinal_lane_refernce_trigger input; T input; Vxo input; Vxt input; ax_max input; jx_max input; Vx output; t output
function [Vx,t] = fcn(longitudinal_lane_refernce_trigger,T,Vxo,Vxt,ax_max,jx_max)
Vx=0;
Ax=0;
t=0;

if Vxt < Vxo
    ax_max=-ax_max;
    jx_max=-jx_max;
end

if longitudinal_lane_refernce_trigger==1

t1=ax_max/jx_max;
t2=(Vxt-Vxo)/ax_max;
t3=t1+t2;
t=T+0.1;


V1=Vxo+(0.5*jx_max*(t1^2));
V2=V1+(ax_max*(t2-t1));
   if t>=0 && t<=t1
       Ax=jx_max*t;
       Vx=double(Vxo+0.5*jx_max*(t^2));
   end
   if t>t1 && t<=t2
       Ax=ax_max;
       Vx=double(V1+(ax_max*(t-t1)));
   end
   if t>t2 && t<=t3
       Ax=ax_max-(jx_max*(t-t2));
       Vx=double(V2+ax_max*(t-t2)-0.5*jx_max*((t-t2)^2));
   end
   if t>t3
       Vx=double(Vxt);
       Ax=0;
   end
       

end
if longitudinal_lane_refernce_trigger==0
  Vx=double(Vxo);
 

   
end
end

== matlab function acc_with_sensor/Subsystem/longitudinal_driver_reference4 ==
  data: longitudinal_lane_refernce_trigger input; T input; Vxo input; Vxt input; ax_max input; jx_max input; Vx output; t output
function [Vx,t] = fcn(longitudinal_lane_refernce_trigger,T,Vxo,Vxt,ax_max,jx_max)
Vx=0;
Ax=0;
t=0;

if Vxt < Vxo
    ax_max=-ax_max;
    jx_max=-jx_max;
end

if longitudinal_lane_refernce_trigger==1

t1=ax_max/jx_max;
t2=(Vxt-Vxo)/ax_max;
t3=t1+t2;
t=T+0.1;


V1=Vxo+(0.5*jx_max*(t1^2));
V2=V1+(ax_max*(t2-t1));
   if t>=0 && t<=t1
       Ax=jx_max*t;
       Vx=double(Vxo+0.5*jx_max*(t^2));
   end
   if t>t1 && t<=t2
       Ax=ax_max;
       Vx=double(V1+(ax_max*(t-t1)));
   end
   if t>t2 && t<=t3
       Ax=ax_max-(jx_max*(t-t2));
       Vx=double(V2+ax_max*(t-t2)-0.5*jx_max*((t-t2)^2));
   end
   if t>t3
       Vx=double(Vxt);
       Ax=0;
   end
       

end
if longitudinal_lane_refernce_trigger==0
  Vx=double(Vxo);
 

   
end
end

== matlab function acc_with_sensor/Subsystem/longitudinal_driver_reference5 ==
  data: longitudinal_lane_refernce_trigger input; T input; Vxo input; Vxt input; ax_max input; jx_max input; Vx output; t output
function [Vx,t] = fcn(longitudinal_lane_refernce_trigger,T,Vxo,Vxt,ax_max,jx_max)
Vx=0;
Ax=0;
t=0;

if Vxt < Vxo
    ax_max=-ax_max;
    jx_max=-jx_max;
end

if longitudinal_lane_refernce_trigger==1

t1=ax_max/jx_max;
t2=(Vxt-Vxo)/ax_max;
t3=t1+t2;
t=T+0.1;


V1=Vxo+(0.5*jx_max*(t1^2));
V2=V1+(ax_max*(t2-t1));
   if t>=0 && t<=t1
       Ax=jx_max*t;
       Vx=double(Vxo+0.5*jx_max*(t^2));
   end
   if t>t1 && t<=t2
       Ax=ax_max;
       Vx=double(V1+(ax_max*(t-t1)));
   end
   if t>t2 && t<=t3
       Ax=ax_max-(jx_max*(t-t2));
       Vx=double(V2+ax_max*(t-t2)-0.5*jx_max*((t-t2)^2));
   end
   if t>t3
       Vx=double(Vxt);
       Ax=0;
   end
       

end
if longitudinal_lane_refernce_trigger==0
  Vx=double(Vxo);
 

   
end
end

== matlab function acc_with_sensor/Subsystem/longitudinal_driver_reference6 ==
  data: longitudinal_lane_refernce_trigger input; T input; Vxo input; Vxt input; ax_max input; jx_max input; Vx output; t output
function [Vx,t] = fcn(longitudinal_lane_refernce_trigger,T,Vxo,Vxt,ax_max,jx_max)
Vx=0;
Ax=0;
t=0;

if Vxt < Vxo
    ax_max=-ax_max;
    jx_max=-jx_max;
end

if longitudinal_lane_refernce_trigger==1

t1=ax_max/jx_max;
t2=(Vxt-Vxo)/ax_max;
t3=t1+t2;
t=T+0.1;


V1=Vxo+(0.5*jx_max*(t1^2));
V2=V1+(ax_max*(t2-t1));
   if t>=0 && t<=t1
       Ax=jx_max*t;
       Vx=double(Vxo+0.5*jx_max*(t^2));
   end
   if t>t1 && t<=t2
       Ax=ax_max;
       Vx=double(V1+(ax_max*(t-t1)));
   end
   if t>t2 && t<=t3
       Ax=ax_max-(jx_max*(t-t2));
       Vx=double(V2+ax_max*(t-t2)-0.5*jx_max*((t-t2)^2));
   end
   if t>t3
       Vx=double(Vxt);
       Ax=0;
   end
       

end
if longitudinal_lane_refernce_trigger==0
  Vx=double(Vxo);
 

   
end
end

== matlab function acc_with_sensor/Subsystem/longitudinal_driver_reference7 ==
  data: longitudinal_lane_refernce_trigger input; T input; Vxo input; Vxt input; ax_max input; jx_max input; Vx output; t output
function [Vx,t] = fcn(longitudinal_lane_refernce_trigger,T,Vxo,Vxt,ax_max,jx_max)
Vx=0;
Ax=0;
t=0;

if Vxt < Vxo
    ax_max=-ax_max;
    jx_max=-jx_max;
end

if longitudinal_lane_refernce_trigger==1

t1=ax_max/jx_max;
t2=(Vxt-Vxo)/ax_max;
t3=t1+t2;
t=T+0.1;


V1=Vxo+(0.5*jx_max*(t1^2));
V2=V1+(ax_max*(t2-t1));
   if t>=0 && t<=t1
       Ax=jx_max*t;
       Vx=double(Vxo+0.5*jx_max*(t^2));
   end
   if t>t1 && t<=t2
       Ax=ax_max;
       Vx=double(V1+(ax_max*(t-t1)));
   end
   if t>t2 && t<=t3
       Ax=ax_max-(jx_max*(t-t2));
       Vx=double(V2+ax_max*(t-t2)-0.5*jx_max*((t-t2)^2));
   end
   if t>t3
       Vx=double(Vxt);
       Ax=0;
   end
       

end
if longitudinal_lane_refernce_trigger==0
  Vx=double(Vxo);
 

   
end
end
